simulink subsystem "coders"  (R2022b)
settings: Solver=VariableStepAuto  StartTime=0.0  StopTime=10.0  RelTol=1e-3
settings Model: Creator=LeonK  LastModifiedBy=LeonK

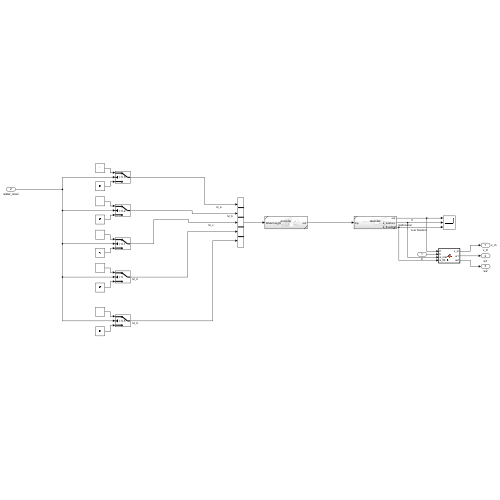
[thumbnail: Simulink's stored preview of the top-level diagram]
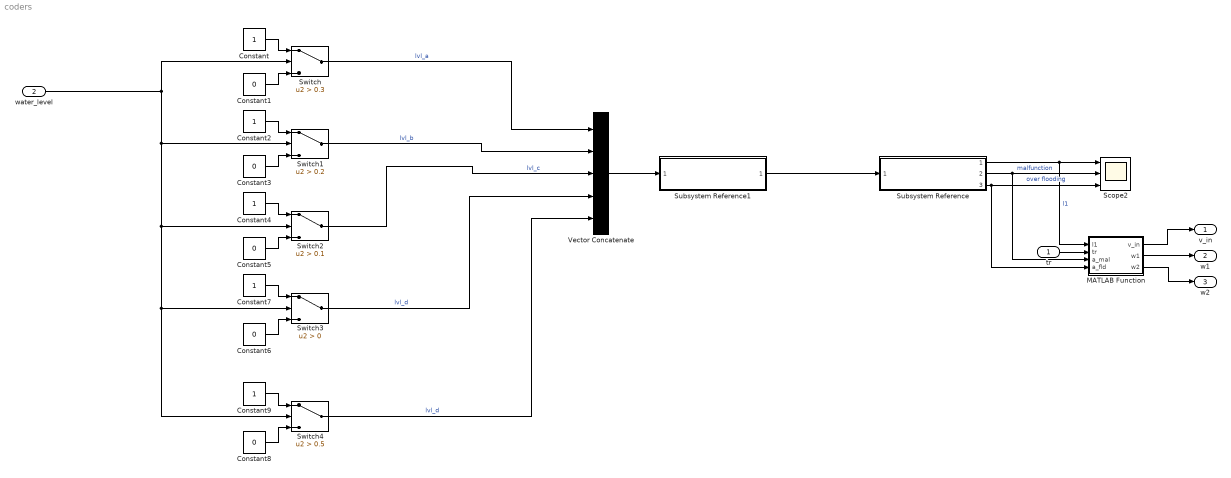
== system coders ==
  tr : Inport
  water_level : Inport  Port=2
  Constant{,2,4,7,9} (5 alike) : Constant
  Constant{1,3,5..6,8} (5 alike) : Constant  Value=0
  MATLAB Function : MATLAB Function  TreatAsAtomicUnit=on
  Scope2 : Scope  NumInputPorts=3
  Subsystem Reference : Subsystem  ReferencedSubsystem=decoder
  Subsystem Reference1 : Subsystem  ReferencedSubsystem=encoder
  Switch : Switch  Criteria=u2 > Threshold  Threshold=0.3  SaturateOnIntegerOverflow=off  InputSameDT=off
  Switch1 : Switch  Criteria=u2 > Threshold  Threshold=0.2  SaturateOnIntegerOverflow=off  InputSameDT=off
  Switch2 : Switch  Criteria=u2 > Threshold  Threshold=0.1  SaturateOnIntegerOverflow=off  InputSameDT=off
  Switch3 : Switch  Criteria=u2 > Threshold  SaturateOnIntegerOverflow=off  InputSameDT=off
  Switch4 : Switch  Criteria=u2 > Threshold  Threshold=0.5  SaturateOnIntegerOverflow=off  InputSameDT=off
  Vector Concatenate : Concatenate  NumInputs=5
  v_in : Outport  SignalName=v_in
  w1 : Outport  Port=2
  w2 : Outport  Port=3
  wires:
  tr/1 -> MATLAB Function/2(tr)
  MATLAB Function/3(w2) -> w2/1
  Subsystem Reference/2 -> MATLAB Function/3(a_mal), Scope2/2  "malfunction"
  MATLAB Function/1(v_in) -> v_in/1
  Subsystem Reference/3 -> MATLAB Function/4(a_fld), Scope2/3  "over flooding"
  Subsystem Reference1/1 -> Subsystem Reference/1
  Subsystem Reference/1 -> MATLAB Function/1(l1), Scope2/1  "l1"
  MATLAB Function/2(w1) -> w1/1
  Constant7/1 -> Switch3/1
  Vector Concatenate/1 -> Subsystem Reference1/1
  Switch2/1 -> Vector Concatenate/3  "lvl_c"
  Switch1/1 -> Vector Concatenate/2  "lvl_b"
  Constant3/1 -> Switch1/3
  Constant6/1 -> Switch3/3
  Constant4/1 -> Switch2/1
  water_level/1 -> Switch2/2, Switch4/2, Switch3/2, Switch1/2, Switch/2
  Switch/1 -> Vector Concatenate/1  "lvl_a"
  Constant5/1 -> Switch2/3
  Constant2/1 -> Switch1/1
  Constant1/1 -> Switch/3
  Constant/1 -> Switch/1
  Switch3/1 -> Vector Concatenate/4  "lvl_d"
  Constant9/1 -> Switch4/1
  Constant8/1 -> Switch4/3
  Switch4/1 -> Vector Concatenate/5  "lvl_d"

== matlab function coders/MATLAB Function ==
  data: l1 input; v_in output; tr input; a_mal input; a_fld input; w1 output; w2 output
function [v_in, w1, w2] = fcn(l1, tr, a_mal, a_fld)
    rho = 1; % constant for product with ambient temperature
    if (l1==3)
        v_in = 5;
    elseif (l1==4 || l1==5)
        v_in = 10;
    else
        v_in = 0;
    end
    if (l1>= 2 && tr >= 293 * rho)
        w1 = 1;
    else
        w1 = 0;
    end
    if (a_mal || a_fld || l1 >= 5)
        w2 = 1;
    else
        w2 = 0;
    end
